simulink model "EthernetPC"  (R2015b)
settings: Solver=FixedStepDiscrete  StartTime=0.0  StopTime=inf  FixedStep=0.1  RelTol=1e-3
libraries: xpcutilitieslib x2, instrumentlib x1
settings Model: xpc_rtwmakecfg_data=_xpcnblib__xpcetherlib__xpcether8255xlib__xpcetherGbElib_  Creator=User  LastModifiedBy=Druzhinin_Vasily

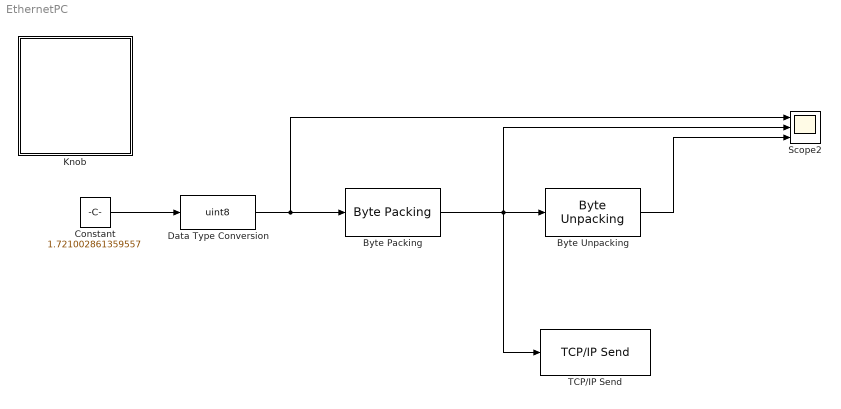
== system EthernetPC ==
  "Byte Packing " : xpcutilitieslib/Byte Packing   MaskPackedDataType=uint8  MaskUnpackedDataTypes={'uint8'}  MaskAlignment=1
  "Byte Unpacking " : xpcutilitieslib/Byte Unpacking   MaskUnpackedDataTypes={'uint8'}  MaskUnpackedDataSizes={[1]}  MaskAlignment=1
  Constant : Constant  Value=1.721002861359557
  Data Type Conversion : DataTypeConversion  OutDataTypeStr=uint8
  Knob : Subsystem  DialogController=hmiCreateDDGDialog  IsWebBlock=on  mask(MWDashboardBlock){webBlockId=431c8b31-2962-49dc-819f-aea9d6f41e3d, webBlockType=continuousknob, ShowInLibBrowser=on, ShowInitialText=on, HMISrcModelName=EthernetPC}
      mask prompts: webBlockId "WebBlock Id"; webBlockType "WebBlock Type"; HMISrcModelName "Source Model"
      mask Help: helpview([docroot '/mapfiles/simulink.map'], 'hmi_knob')
      mask Display:
      | if strcmp(get_param(bdroot(gcb),'BlockDiagramType'), 'library')
      |     image([(matlabroot) '/toolbox/simulink/hmi/icons/ContinuousKnob.png']);
      | end
  Scope2 : Scope  NumInputPorts=3
  TCP/IP Send : instrumentlib/TCP//IP Send  Host=192.168.110.198  Port=5896  EnableBlockingMode=on  Timeout=1  ByteOrder=BigEndian
  wires:
  Constant/1 -> Data Type Conversion/1
  Data Type Conversion/1 -> Scope2/1, "Byte Packing "/1
  "Byte Unpacking "/1 -> Scope2/3
  "Byte Packing "/1 -> TCP/IP Send/1, Scope2/2, "Byte Unpacking "/1

== system EthernetPC/Knob ==
